simulink model "Buck_Boost__Ser"  (R2020b)
settings: Solver=ode23tb  StartTime=0.0  StopTime=3  RelTol=1e-3
values from neighbouring files (symbols this model uses):
  C = 2200e-6    (= 0.0022)    [Parameters.m]    (also in Parameters_Buck_Boost.m = 0.00022; boost.m = 0.00022)
  d = 0.5    [Parameters.m]    (also in Parameters_Buck_Boost.m; boost.m)
  f = 5000    [Parameters.m]    (also in Parameters_Buck_Boost.m; boost.m)
  L = 820e-6    (= 0.00082)    [Parameters.m]    (also in Parameters_Buck_Boost.m = 0.0008; boost.m = 0.0008)
  R = 50    [Parameters.m]    (also in Parameters_Buck_Boost.m = 7; boost.m = 7)
  Vin = 5    [Parameters.m]    (also in Parameters_Buck_Boost.m = 14; boost.m = 14)
libraries: powerlib x19, powerlib_meascontrol x4
settings Model: Creator=ashka  LastModifiedBy=ashka

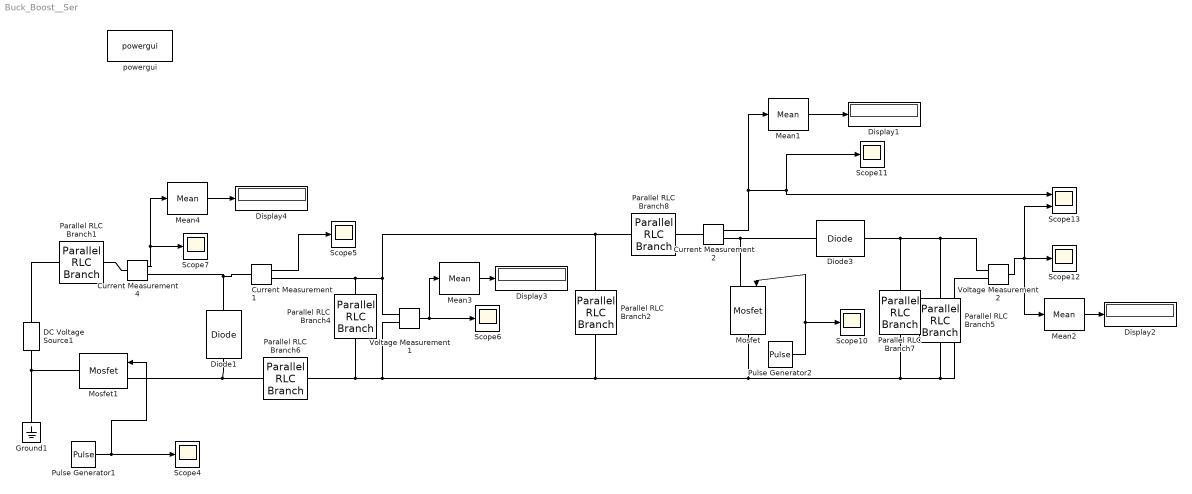
== system Buck_Boost__Ser ==
  Current Measurement1 : powerlib/Measurements/Current Measurement  PhasorSimulation=off  OutputType=Complex  PSBequivalent=0
  Current Measurement2 : powerlib/Measurements/Current Measurement  PhasorSimulation=off  OutputType=Complex  PSBequivalent=0
  Current Measurement4 : powerlib/Measurements/Current Measurement  PhasorSimulation=off  OutputType=Complex  PSBequivalent=0
  DC Voltage Source1 : powerlib/Electrical Sources/DC Voltage Source  Amplitude=Vin  Measurements=None
  Diode1 : powerlib/Power Electronics/Diode  Ron=0.001  Lon=0  Vf=0.8  IC=0  UseSnubber=0  Rs=500  Cs=250e-9  Measurements=off
  Diode3 : powerlib/Power Electronics/Diode  Ron=0.001  Lon=0  Vf=0.8  IC=0  UseSnubber=0  Rs=500  Cs=250e-9  Measurements=off
  Display{1..4} (4 alike) : Display
  Ground1 : powerlib/Elements/Ground  LConnTagsString=a
  Mean1 : powerlib_meascontrol/Measurements/Mean  Freq=f  Vinit=0  Ts=0
  Mean2 : powerlib_meascontrol/Measurements/Mean  Freq=f  Vinit=0  Ts=0
  Mean3 : powerlib_meascontrol/Measurements/Mean  Freq=f  Vinit=7  Ts=0
  Mean4 : powerlib_meascontrol/Measurements/Mean  Freq=f  Vinit=0  Ts=0
  Mosfet : powerlib/Power Electronics/Mosfet  Ron=0.1  Lon=0  Rd=0.01  Vfd=0  IC=0  Rs=1e5  Cs=inf  Measurements=off
  Mosfet1 : powerlib/Power Electronics/Mosfet  Ron=0.1  Lon=0  Rd=0.01  Vfd=0  IC=0  Rs=1e5  Cs=inf  Measurements=off
  Parallel RLC Branch1 : powerlib/Elements/Parallel RLC Branch  LConnTagsString=a  RConnTagsString=__new0  BranchType=R  Resistance=0.001  Inductance=10e-3  SetiL0=off  InitialCurrent=0  Capacitance=1e-6  Setx0=off  InitialVoltage=0  Measurements=None
  Parallel RLC Branch2 : powerlib/Elements/Parallel RLC Branch  LConnTagsString=a  RConnTagsString=__new0  BranchType=C  Resistance=R  Inductance=10e-3  SetiL0=off  InitialCurrent=0  Capacitance=1  Setx0=off  InitialVoltage=0  Measurements=None
  Parallel RLC Branch4 : powerlib/Elements/Parallel RLC Branch  LConnTagsString=a  RConnTagsString=__new0  BranchType=C  Resistance=10  Inductance=1e-3  SetiL0=off  InitialCurrent=0  Capacitance=C  Setx0=off  InitialVoltage=0  Measurements=None
  Parallel RLC Branch5 : powerlib/Elements/Parallel RLC Branch  LConnTagsString=a  RConnTagsString=__new0  BranchType=R  Resistance=R  Inductance=10e-3  SetiL0=off  InitialCurrent=0  Capacitance=1e-6  Setx0=off  InitialVoltage=0  Measurements=None
  Parallel RLC Branch6 : powerlib/Elements/Parallel RLC Branch  LConnTagsString=a  RConnTagsString=__new0  BranchType=L  Resistance=10  Inductance=L  SetiL0=off  InitialCurrent=0  Capacitance=1e-6  Setx0=off  InitialVoltage=0  Measurements=None
  Parallel RLC Branch7 : powerlib/Elements/Parallel RLC Branch  LConnTagsString=a  RConnTagsString=__new0  BranchType=C  Resistance=10  Inductance=1e-3  SetiL0=off  InitialCurrent=0  Capacitance=C  Setx0=off  InitialVoltage=0  Measurements=None
  Parallel RLC Branch8 : powerlib/Elements/Parallel RLC Branch  LConnTagsString=a  RConnTagsString=__new0  BranchType=L  Resistance=10  Inductance=L  SetiL0=off  InitialCurrent=0  Capacitance=1e-6  Setx0=off  InitialVoltage=0  Measurements=None
  Pulse Generator1 : DiscretePulseGenerator  PulseType=Time based  Amplitude=10  Period=1/f  PulseWidth=d*100
  Pulse Generator2 : DiscretePulseGenerator  PulseType=Time based  Amplitude=10  Period=1/f  PulseWidth=d*100
  Scope{4..7,10..12} (7 alike) : Scope
  Scope13 : Scope  NumInputPorts=2
  Voltage Measurement1 : powerlib/Measurements/Voltage Measurement  PhasorSimulation=off  OutputType=Complex  PSBequivalent=0
  Voltage Measurement2 : powerlib/Measurements/Voltage Measurement  PhasorSimulation=off  OutputType=Complex  PSBequivalent=0
  powergui : powerlib/powergui  Priority=1  SimulationMode=Continuous  SampleTime=50e-6  frequency=60  Iterations=50  frequencyindice=0  Pbase=100e6  ErrMax=1e-4  UnitsV=kV  UnitsW=MW  buscounter=0  FunctionMessages=off  echomessages=off  EnableUseOfTLC=off  CurrentSourceSwitches=off  DisableSnubberDevices=off  DisableRonSwitches=off  DisableVfSwitches=off  DisplayEquations=off  AutomaticDiscreteSolvers=off  SolverType=Tustin/Backward Euler (TBE)  Interpol=off  ExternalGateDelay=off  methode=off  Ts=100  x0status=blocks  SPID=on  SwTol=0  HookPort=off  NonlinearTolerance=1e-4  nMaxIteration=100  ContinueOnMaxIteration=off  RestoreLinks=warning  ResistiveCurrentMeasurement=off  Frange=[0:2:500]  Ylog=off  Xlog=on  ShowGrid=off  save=off  variable=ZData  structure=0  ZoomFFT=off  StartTime=0.0  cycles=1  DisplayStyle=1  fundamental=60  FreqAxis=off  MaxFrequency=1000  frequencyindicesteady=1  RmsSteady=1  display=off
  wires:
  Mean2/1 -> Display2/1
  Current Measurement2/1 -> Scope11/1, Scope13/1, Mean1/1
  Pulse Generator2/1 -> Scope10/1, Mosfet/1
  Voltage Measurement2/1 -> Scope12/1, Scope13/2, Mean2/1
  Mean1/1 -> Display1/1
  Current Measurement4/1 -> Mean4/1, Scope7/1
  Mean3/1 -> Display3/1
  Voltage Measurement1/1 -> Scope6/1, Mean3/1
  Pulse Generator1/1 -> Mosfet1/1, Scope4/1
  Current Measurement1/1 -> Scope5/1
  Mean4/1 -> Display4/1
  connections:
  Parallel RLC Branch7/LConn1 -- Parallel RLC Branch5/LConn1 -- Voltage Measurement2/LConn1 -- Diode3/RConn1
  Mosfet/LConn1 -- Diode3/LConn1 -- Current Measurement2/RConn1
  Parallel RLC Branch8/LConn1 -- Current Measurement2/LConn1
  Parallel RLC Branch4/LConn1 -- Parallel RLC Branch8/RConn1 -- Parallel RLC Branch2/LConn1 -- Voltage Measurement1/LConn1 -- Current Measurement1/RConn1
  Current Measurement1/LConn1 -- Diode1/RConn1 -- Current Measurement4/RConn1
  Parallel RLC Branch4/RConn1 -- Parallel RLC Branch5/RConn1 -- Voltage Measurement2/LConn2 -- Parallel RLC Branch7/RConn1 -- Mosfet/RConn1 -- Parallel RLC Branch2/RConn1 -- Voltage Measurement1/LConn2 -- Parallel RLC Branch6/LConn1
  DC Voltage Source1/LConn1 -- Ground1/LConn1 -- Mosfet1/RConn1
  Mosfet1/LConn1 -- Parallel RLC Branch6/RConn1 -- Diode1/LConn1
  Parallel RLC Branch1/LConn1 -- Current Measurement4/LConn1
  DC Voltage Source1/RConn1 -- Parallel RLC Branch1/RConn1
